simulink model "NavFilterTestHarness24"  (Simulink 7.9)
settings: Solver=FixedStepDiscrete  StartTime=min(IMUtime)  StopTime=max(IMUtime)  FixedStep=0.001  RelTol=1e-3
undefined symbols (not defined in the file or in its folder): accel, ADSframe, ADStime, angRate, ATTframe, CourseDeg, GndSpd, GPSframe, GPStime, Hgt, IMUframe, IMUtime, LatDeg, LngDeg, MagBiasX, MagBiasY, MagBiasZ, MAGframe, MAGtime, MagX, MagY, MagZ, Pitch, Roll, Veas, VelD, Yaw
libraries: simulink x15
(part 5 of 5)

== matlab function InertialNavFilter/Store States at GPS Meas Time ==
  data: FuseData output double; States input double; measDataArrived input double; StatesAtMeasTime output double; Ndelay input double; ratio input double
%#codegen
function [FuseData,StatesAtMeasTime]   = StoreStatesAtMeasTime(States,measDataArrived,Ndelay,ratio)

% Implement a state sampler that stores the state inoput from Ndelay 
% samples before the measurement is predicted to arrive. When the
% measurement arrives, the stored state is output along with a data fusion
% request. This enables the filter to account for lag in sensors that can
% in some cases be greater than 1 measurement time step. the delay time si
% specified in units of the state prediction delta time. For example if a 
% delay of 0.16 seconds was required, and the state prediction ran at 50 Hz
% then Ndelay would be set to 50*0.15 = 8.
% It is assumed that this function is called the same rate as the state 
% prediction, and that the measurement data comes in at a constant
% rate.
% The 'ratio'specifies the ratio of the state prediction to measurement
% data rates. For example if the state prediction occurres at 50Hz and the
% measurements are being received at 5Hz, then 'ratio' = 50/5 = 10

% This function avoids the need to use large data buffers
% It is generic function that can be used for states required by all
% measurement fusion processes, and as such has not been optimised to only
% includes the specific states required, or the buffer arry length trimmed
% to the minimum required.

% Ndelay cannot be zero and cannot exceed a value of 10*ratio-1
Ndelay = max(min(Ndelay,int32(10*ratio)),int32(1));

majorStepDelay = int32(ceil(single(Ndelay)/single(ratio)));
minorStepDelay = int32(rem(single(Ndelay),single(ratio)));

persistent prevStatesMatrix;
if isempty(prevStatesMatrix)
    prevStatesMatrix = single(zeros(24,11));
end

persistent totalFrameCount;
if isempty(totalFrameCount)
    totalFrameCount = int32(0);
end

persistent measID;
if isempty(measID)
    measID = int32(zeros(1,11));
end

persistent minorFrameCount;
if isempty(minorFrameCount)
    minorFrameCount = int32(0);
end

totalFrameCount = totalFrameCount + int32(1);
minorFrameCount = minorFrameCount + int32(1);

if measDataArrived
    if measID(1) ~= 0
        FuseData = logical(1);
    else
        FuseData = logical(0);
    end
    if abs(single(totalFrameCount - measID(1) - Ndelay)) < 0.5*single(ratio)
        StatesAtMeasTime = prevStatesMatrix(:,1);
    else
        frameErrors = abs(measID - totalFrameCount + Ndelay);
        bestError = Ndelay;
        bestIndex = int32(1);
        for index = 1:majorStepDelay
            if frameErrors(index) < bestError
                bestError = frameErrors(index);
                bestIndex = index;
            end
        end
        StatesAtMeasTime = prevStatesMatrix(:,bestIndex);
    end
else
    StatesAtMeasTime = single(zeros(24,1));
    FuseData = logical(0);
end

if minorFrameCount == (ratio - minorStepDelay)
    if majorStepDelay > int32(0)
        for index = 1:majorStepDelay
            prevStatesMatrix(:,index) = prevStatesMatrix(:,index+1);
            measID(index) = measID(index+1);
        end
    end
    prevStatesMatrix(:,majorStepDelay) = States;
    measID(majorStepDelay) = totalFrameCount;
end

if measDataArrived
    minorFrameCount = int32(0);
end

end

== matlab function InertialNavFilter/Read Measurements/Convert GPS Data ==
  data: VelNED output double; PosNE output double; GPS_DataArrived input double; RefLatLongDeg input double; LatLongDeg input double; GndSpd input double; CourseDeg input double; VelD input double
%#codegen
function [VelNED,PosNE]   = ConvertGpsData(GPS_DataArrived,RefLatLongDeg,LatLongDeg,GndSpd,CourseDeg,VelD)

% Do a conversion from lat,long to local North.Est position relative to a
% reference point using WGS-84 eaerth radius and using a simple spherical
% earth model
% Convert GPS course and speed to North and East velocity components

deg2rad = single(pi/180);
earthRadius = single(6378145);

PosNE = single(zeros(2,1));
VelNED = single(zeros(3,1));
LatLongDelta = (LatLongDeg-RefLatLongDeg) * deg2rad;
PosNE(1) = earthRadius * LatLongDelta(1);
PosNE(2) = earthRadius * cos(RefLatLongDeg(1)*deg2rad) * LatLongDelta(2);
VelNED(1) = GndSpd*cos(CourseDeg*deg2rad);
VelNED(2) = GndSpd*sin(CourseDeg*deg2rad);
VelNED(3) = VelD;

return

== matlab function InertialNavFilter/Read Measurements/Calculate Delta Angles & Velocities ==
  data: delAngIMU output double; delVelIMU output double; angRateIMU input double; accelIMU input double; dtIMU input double
%#codegen
function [delAngIMU,delVelIMU]  = CalcDeltaAngVel(angRateIMU, accelIMU, dtIMU)

persistent prevAngRateIMU;
if isempty(prevAngRateIMU)
    prevAngRateIMU = single([0;0;0]);
end
persistent prevAccelIMU;
if isempty(prevAccelIMU)
    prevAccelIMU = single([0;0;0]);
end

% Apply trapezoidal integration
delAngIMU = 0.5*dtIMU*(angRateIMU + prevAngRateIMU);
delVelIMU = 0.5*dtIMU*(accelIMU   + prevAccelIMU  );

prevAngRateIMU = angRateIMU;
prevAccelIMU   = accelIMU;

end

== matlab function InertialNavFilter/Fuse Vel Pos Measurements ==
  data: states input double; P input double; accNavMag input double; FuseGPSData input double; VelNED input double; PosNE input double; StatesAtGpsTime input double; FuseHgtData input double; HgtMea input double; nextStates output double; nextP output double; innovation output double; varInnov output double; StatesAtHgtTime input double; useAirspeed input double
%#codegen
function [...
    nextStates, ... % state vector after fusion of measurements (q0, ... , q3, VelN,E,D, PosN,E,D, WindN,E, P0, camera roll pitch yaw misalignment)
    nextP, ... % state covariance matrix after fusion of corrections
    innovation,... % NED velocity and NED position innovations (m/s, m)
    varInnov] ... % NED velocity and NED position innovation variance ((m/s)^2, m^2)
    = FuseVelPosNED( ...
    states, ... % predicted states from the INS (q0, ... , q3, VelN,E,D, PosN,E,D, WindN,E, P0, camera roll pitch yaw misalignment)
    P, ... % predicted covariance
    accNavMag, ... % magnitude of rate of change of velocity in navigation frame (m/s^2)
    FuseGPSData, ... % Boolean to initiate fusion of GPS measurements
    VelNED, ... % NED velocity measurements (m/s)
    PosNE, ... % NE position measurements (m)
    StatesAtGpsTime, ... % States captured at GPs measurement time
    FuseHgtData, ... % Boolean to initiate fusion of height measurements
    HgtMea, ... % D position measurement (m)
    StatesAtHgtTime, ... % States captured at height measurement time
    useAirspeed) % Boolean to indicate that an airspeed sensor is being used

% define persistent variables
persistent velFailCount;
if isempty(velFailCount)
    velFailCount = uint32(0);
end
persistent posFailCount;
if isempty(posFailCount)
    posFailCount = uint32(0);
end
persistent hgtFailCount;
if isempty(hgtFailCount)
    hgtFailCount = uint32(0);
end

% initialise measurement health flags to false
velHealth = 0;
posHealth = 0;
hgtHealth = 0;

% Specify GPS velocity induced error
velErr = single(0.15*accNavMag);
posErr = single(0.15*accNavMag);
% Specify the GPS and height measurement variances.
R_OBS = single([(0.1^2 + velErr^2) (0.1^2 + velErr^2) (0.1^2 + velErr^2) (2.0^2 + posErr^2) (2.0^2 + posErr^2) 2.0^2]);

% Specify the count before forcing use of GPS or height data after invalid
% data. We need to force GPS again sooner without
% airspeed data as the nav velocities will be unconstrained.
gpsRetryTime = single(30);
gpsRetryTimeNoTAS = single(5);
hgtRetryTime = single(30);
dt = single(0.02);
if useAirspeed
    maxVelFailCount = round(gpsRetryTime/dt);
    maxPosFailCount = maxVelFailCount;
else
    maxVelFailCount = round(gpsRetryTimeNoTAS/dt);
    maxPosFailCount = maxVelFailCount;
end
maxHgtFailCount = round(hgtRetryTime/dt);

% initialise the innovation vector
innovation = single(zeros(6,1));

% initialise the innovation variance vector
varInnov = single(zeros(6,1));

% Define the observation vector
observation = single([VelNED;PosNE;-HgtMea]);

% Perform sequential fusion of GPS measurements. This assumes that the
% errors in the dfferent velocity and position componenets are
% uncorrelated which is not true, however in the absence of covariance
% data from the GPS receiver it is the only assumption we can make
% so we might as well take advantage of the computational efficiencies
% associated with sequential fusion
if (FuseGPSData || FuseHgtData)
    % calculate innovation variances
    for obsIndex = 1:6
        stateIndex = 4 + obsIndex;
        varInnov(obsIndex) = P(stateIndex,stateIndex) + R_OBS(obsIndex);
    end
    % calculate innovations and check validity against limits
    if FuseGPSData
        velInnov = StatesAtGpsTime(5:7) - VelNED;
        if (velInnov(1)*velInnov(1) + velInnov(2)*velInnov(2) + velInnov(3)*velInnov(3)) < 25.0*(varInnov(1) + varInnov(2) + varInnov(3)) || ...
                (velFailCount > maxVelFailCount)
            velHealth = 1;
            velFailCount = uint32(0);
        else
            velHealth = 0;
            velFailCount = velFailCount + uint32(1);
        end
        posInnov = StatesAtGpsTime(8:9) - PosNE;
        if (posInnov(1)*posInnov(1) + posInnov(2)*posInnov(2)) < 100.0*(varInnov(4) + varInnov(5)) || ...
                (posFailCount > maxPosFailCount)
            posHealth = 1;
            posFailCount = uint32(0);
        else
            posHealth = 0;
            posFailCount = posFailCount + uint32(1);
        end
    end
    if FuseHgtData
        hgtInnov = StatesAtHgtTime(10) + HgtMea;
        if (hgtInnov*hgtInnov) < 25.0*varInnov(6) || ...
                (hgtFailCount > maxHgtFailCount)
            hgtHealth = 1;
            hgtFailCount = uint32(0);
        else
            hgtHealth = 0;
            hgtFailCount = hgtFailCount + uint32(1);
        end
    end
    % Set range for sequential fusion of velocity and position measurements
    if FuseGPSData
        startIndex = 1;
    else
        startIndex = 6;
    end
    if FuseHgtData
        endIndex = 6;
    else
        endIndex = 5;
    end
    % Fuse measurements sequentially
    for obsIndex = startIndex:endIndex
        % Apply data health checks
        % If no airspeed data, start using GPS data after x seconds
        if (velHealth && (obsIndex >= 1 && obsIndex <= 3)) || ...
                (posHealth && (obsIndex == 4 || obsIndex == 5)) || ...
                (hgtHealth && (obsIndex == 6))
            stateIndex = 4 + obsIndex;
            % Calculate the measurement innovation, using states from the
            % appropriate time coordinate
            if obsIndex == 6
                innovation(obsIndex) = StatesAtHgtTime(stateIndex) - observation(obsIndex);
            else
                innovation(obsIndex) = StatesAtGpsTime(stateIndex) - observation(obsIndex);
            end
            % Calculate the Kalman Gain
            varInnov(obsIndex) = P(stateIndex,stateIndex) + R_OBS(obsIndex); % data logging only
            SK = 1/varInnov(obsIndex);
            K = P(:,stateIndex)*SK;
            % Calculate state corrections
            xk = K * innovation(obsIndex);
            % Update the covariance - take advantage of direct observation of a
            % single state at stateIndex
            %P = (I - K*H)*P;
            KHP = single(zeros(24,24));
            for rowIndex = 1:24
                for colIndex = 1:24
                    KHP(rowIndex,colIndex) = K(rowIndex)*P(stateIndex,colIndex);
                end
            end
            P = P - KHP;
            % Apply the state corrections and re-normaliase the quaternions
            states = states - xk;
            % Normalise the quaternion states
            quatMag = sqrt(states(1)^2 + states(2)^2 + states(3)^2 + states(4)^2);
            if (quatMag > 1e-12)
                states(1:4) = states(1:4) / quatMag;
            end
        end
    end
end
% Output covariance matrix and state vector
nextP = P;
nextStates = states;
end
